simulink model "AWD_EV_MODEL_rev2"  (Simulink 8.7)
settings: Solver=ode3  SolverMode=SingleTasking  StartTime=0.0  StopTime=25  FixedStep=0.001  RelTol=1e-3
undefined symbols (not defined in the file): Bx, Bx_2, By, By_2, Cx, Cx_2, Cy, Cy_2, Dx, Dx_2, Dy, Dy_2, Ex, Ex_2, Ey, Ey_2, g, GRR, GRR_E, hg, Jw, Jz, Lf, Lr, Lw, m, r0, Rw, rx1, rx1_2, rx2, rx2_2, ry1, ry1_2, ry2, ry2_2, sigbuilder_block, Vx0, Vy0, wRL0
libraries: simulink x3
settings Model: Creator=ETLAB  LastModifiedBy=kschmutz
settings SolverCC: AlgebraicLoopSolver=LineSearch
settings DataIOCC: SignalLoggingSaveFormat=ModelDataLogs
settings OptimizationCC: ExpressionDepthLimit=2147483647
settings DebuggingCC: SolverPrmCheckMsg=warning  InheritedTsInSrcMsg=none  FcnCallInpInsideContextMsg=EnableAllAsWarning  StateNameClashWarn=warning
settings GRTTargetCC: CombineOutputUpdateFcns=off  GRTInterface=on

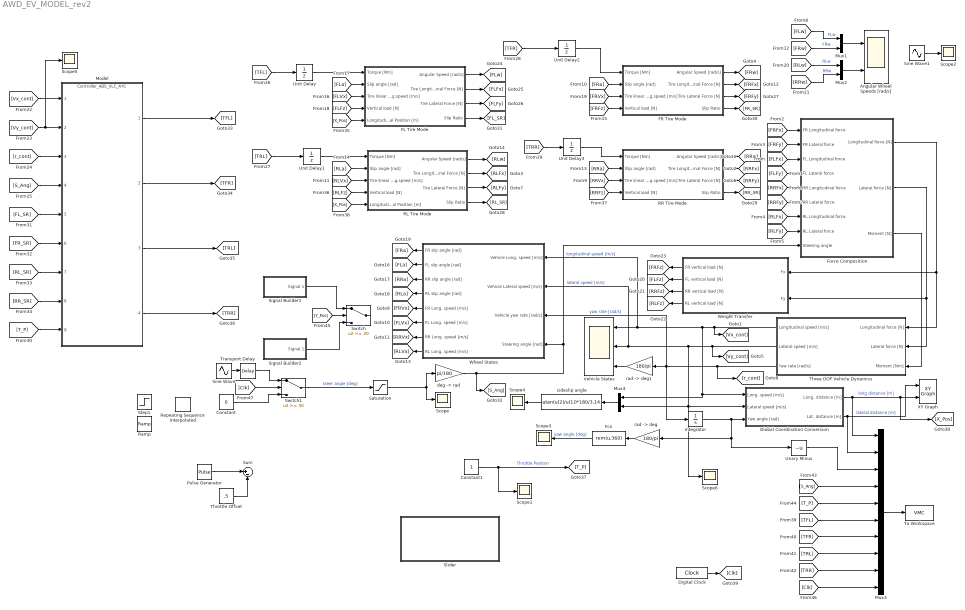
== system AWD_EV_MODEL_rev2 ==
  Angular Wheel Speeds [rad/s] : Scope  NumInputPorts=2
  Constant : Constant  Value=0
  Constant1 : Constant
  Digital Clock : DigitalClock  SampleTime=0.001
  FL Tire Mode : Subsystem
      mask Display:
      | image(imread('Tire.bmp'),'center')
      | port_label('input', 1, 'Torque [Nm]')
      | port_label('input', 2, 'Slip angle [rad]')
      | port_label('input', 3, 'Long. speed [m/s]')
      | port_label('input', 4, 'Vertical load [N]')
      | port_label('input', 5, 'Longitudinal Pos [m]')
      | port_label('output', 1, 'Angular speed [rad/s]')
      | port_label('output', 2, 'Long. force [N]')
      | port_label('output', 3, 'Lateral force [N]')
      | port_label('output', 4, 'Slip Ratio')
  FR Tire Mode : Subsystem
      mask Display:
      | image(imread('Tire.bmp'),'center')
      | port_label('input', 1, 'Torque [Nm]')
      | port_label('input', 2, 'Slip angle [rad]')
      | port_label('input', 3, 'Long. speed [m/s]')
      | port_label('input', 4, 'Vertical load [N]')
      | port_label('output', 1, 'Angular speed [rad/s]')
      | port_label('output', 2, 'Long. force [N]')
      | port_label('output', 3, 'Lateral force [N]')
      | port_label('output', 4, 'Slip Ratio')
  Fcn : Fcn  Expr=rem(u,360)
  Force Composition : Subsystem
  Global Coordination Conversion : Subsystem
  Integrator : Integrator
  Model : ModelReference  ModelNameDialog=Controller_ABS_VLC_AYC  SimulationMode=Normal  ModelReferenceVersion=1.127
  Mux1 : Mux  Inputs=2
  Mux2 : Mux  Inputs=2
  Mux3 : Mux  Inputs=10
  Mux4 : Mux  Inputs=2
  Pulse Generator : DiscretePulseGenerator  PulseType=Time based  Amplitude=.5  Period=7  PulseWidth=50
  RL Tire Mode : Subsystem
      mask Display:
      | image(imread('Tire.bmp'),'center')
      | port_label('input', 1, 'Torque [Nm]')
      | port_label('input', 2, 'Slip angle [rad]')
      | port_label('input', 3, 'Long. speed [m/s]')
      | port_label('input', 4, 'Vertical load [N]')
      | port_label('input', 5, 'Longitudinal Pos [m]')
      | port_label('output', 1, 'Angular speed [rad/s]')
      | port_label('output', 2, 'Long. force [N]')
      | port_label('output', 3, 'Lateral force [N]')
      | port_label('output', 4, 'Slip Ratio')
  RR Tire Mode : Subsystem
      mask Display:
      | image(imread('Tire.bmp'),'center')
      | port_label('input', 1, 'Torque [Nm]')
      | port_label('input', 2, 'Slip angle [rad]')
      | port_label('input', 3, 'Long. speed [m/s]')
      | port_label('input', 4, 'Vertical load [N]')
      | port_label('output', 1, 'Angular speed [rad/s]')
      | port_label('output', 2, 'Long. force [N]')
      | port_label('output', 3, 'Lateral force [N]')
  Ramp : simulink/Sources/Ramp  slope=0  start=.2  X0=0
  Repeating Sequence Interpolated : simulink/Sources/Repeating Sequence Interpolated  OutValues=[0 0 7 0 0 -7 0 0].'  TimeValues=[0 2 4 6 8 10 26 28].'  LookUpMeth=Interpolation-Use End Values  tsamp=0.001  OutMin=[]  OutMax=[]  OutDataTypeStr=double  OutputDataTypeScalingMode=double  OutDataType=fixdt(0,8)  OutScaling=2^-10
  Saturation : Saturate  UpperLimit=15  LowerLimit=-15
  Scope{,1..6} (7 alike) : Scope
  Signal Builder1 : Subsystem  Tag=STV Subsys  LoadFcn=sigbuilder_block('load');  StartFcn=sigbuilder_block('start');  StopFcn=sigbuilder_block('stop');  ClipboardFcn=sigbuilder_block('clipboard');  mask(Sigbuilder block){}
      mask help: Simulink:masks:SigbuilderBlock_MD
      mask init:
      | if ~strcmp(get_param(bdroot(gcbh),'SimulationStatus'),'stopped') tuvar = sigbuilder_block('maskInit'); end
      settings: CopyFcn=sigbuilder_block('copy');  DeleteFcn=sigbuilder_block('delete');  ModelCloseFcn=sigbuilder_block('modelClose');  PreSaveFcn=sigbuilder_block('preSave');  PauseFcn=sigbuilder_block('pause');  ContinueFcn=sigbuilder_block('continue');  NameChangeFcn=sigbuilder_block('namechange');  OpenFcn=sigbuilder_block('open',[6 36 1428 711 ]);  CloseFcn=sigbuilder_block('close');
      mask Display: plot(0, 0, 100, 100,[2, 2, 32, 32, 2], [68, 8, 8, 68, 68],[32, 2], [38, 38], [32, 19, 2],[53, 60, 44], [32, 17, 17, 2],[16, 16, 31, 31]);txt = getActiveGroup(gcbh);text(2, 100, txt,'verticalAlignment', 'top');
  Signal Builder2 : Subsystem  Tag=STV Subsys  LoadFcn=sigbuilder_block('load');  StartFcn=sigbuilder_block('start');  StopFcn=sigbuilder_block('stop');  ClipboardFcn=sigbuilder_block('clipboard');  mask(Sigbuilder block){}
      mask help: Simulink:masks:SigbuilderBlock_MD
      mask init:
      | if ~strcmp(get_param(bdroot(gcbh),'SimulationStatus'),'stopped') tuvar = sigbuilder_block('maskInit'); end
      settings: CopyFcn=sigbuilder_block('copy');  DeleteFcn=sigbuilder_block('delete');  ModelCloseFcn=sigbuilder_block('modelClose');  PreSaveFcn=sigbuilder_block('preSave');  PauseFcn=sigbuilder_block('pause');  ContinueFcn=sigbuilder_block('continue');  NameChangeFcn=sigbuilder_block('namechange');  OpenFcn=sigbuilder_block('open',[6 36 1428 711 ]);  CloseFcn=sigbuilder_block('close');
      mask Display: plot(0, 0, 100, 100,[2, 2, 32, 32, 2], [68, 8, 8, 68, 68],[32, 2], [38, 38], [32, 19, 2],[53, 60, 44], [32, 17, 17, 2],[16, 16, 31, 31]);txt = getActiveGroup(gcbh);text(2, 100, txt,'verticalAlignment', 'top');
  Sine Wave : Sin  Amplitude=4  Frequency=.1  SampleTime=0
  Sine Wave1 : Sin  Frequency=0.5  SampleTime=0
  Slider : Subsystem  DialogController=hmiCreateDDGDialog  DialogControllerArgs=DataTag4  IsWebBlock=on  mask(MWDashboardBlock){webBlockId=ca84606d-5772-4c84-acb2-69dff7348784, webBlockType=slider, ShowInLibBrowser=on, ShowInitialText=on, HMISrcModelName=AWD_EV_MODEL_rev2}
      mask prompts: webBlockId "WebBlock Id"; webBlockType "WebBlock Type"; HMISrcModelName "Source Model"
      mask Help: helpview([docroot '/mapfiles/simulink.map'], 'hmi_slider')
      mask Display:
      | if strcmp(get_param(bdroot(gcb),'BlockDiagramType'), 'library')
      |     image([(matlabroot) '/toolbox/simulink/hmi/icons/Slider.png']);
      | end
  Step1 : Step  Time=0  After=5  SampleTime=0
  Sum : Sum  Inputs=|+-
  Switch : Switch  Threshold=20
  Switch1 : Switch  Threshold=30
  Three DOF Vehicle Dynamics : Subsystem
      mask Display:
      | image(imread('Vehicle.bmp'),'center')
      | port_label('input', 1, 'Longitudinal force [N]')
      | port_label('input', 2, 'Lateral force [N]')
      | port_label('input', 3, 'Moment [Nm]')
      | port_label('output', 1, 'Longitudinal speed [m/s]')
      | port_label('output', 2, 'Lateral speed [m/s]')
      | port_label('output', 3, 'Yaw rate [rad/s]')
  Throttle Offset : Constant  Value=.5
  To Workspace : ToWorkspace  VariableName=VMC  SampleTime=-1
  Transport Delay : TransportDelay  DelayTime=4
  Unary Minus : UnaryMinus
  Unit Delay{,1..3} (4 alike) : UnitDelay  InitialCondition=1  SampleTime=-1
  Vehicle States : Scope  NumInputPorts=3
  Weight Transfer : Subsystem
  Wheel States : Subsystem
  XY Graph : simulink/Sinks/XY Graph  xmin=-500  xmax=500  ymin=-500  ymax=500  st=-1
  "deg -> rad" : Gain  Gain=pi/180
  "rad -> deg" : Gain  Gain=180/pi
  "rad -> deg1" : Gain  Gain=180/pi
  sideslip angle : Fcn  Expr=atan(u(2)/u(1))*180/3.14
  wires:
  Wheel States/5(FR Long. speed [m/s]) -> [FRVx]
  Wheel States/6(FL Long. speed [m/s]) -> [FLVx]
  Wheel States/7(RR Long. speed [m/s]) -> [RRVx]
  Wheel States/8(RL Long. speed [m/s]) -> [RLVx]
  Three DOF Vehicle Dynamics/3(Yaw rate [rad/s]) -> "rad -> deg1"/1, Wheel States/3(Vehicle yaw rate [rad/s]), Integrator/1, [r_cont]  "yaw rate [rad/s]"
  Three DOF Vehicle Dynamics/2(Lateral speed [m/s]) -> Wheel States/2(Vehicle Lateral speed [m/s]), Vehicle States/2, Global Coordination Conversion/2(Lateral speed [m/s]), Mux4/2, Scope6/1, [Vy_cont]  "lateral speed [m/s]"
  Three DOF Vehicle Dynamics/1(Longitudinal speed [m/s]) -> Wheel States/1(Vehicle Long. speed [m/s]), Vehicle States/1, Global Coordination Conversion/1(Long. speed [m/s]), Mux4/1, [Vx_cont]  "longitudinal speed [m/s]"
  Wheel States/1("FR slip angle [rad] ") -> [FRa]
  Wheel States/2("FL slip angle [rad] ") -> [FLa]
  Wheel States/3("RR slip angle [rad] ") -> [RRa]
  Wheel States/4("RL slip angle [rad] ") -> [RLa]
  Force Composition/1(Longitudinal force [N]) -> Weight Transfer/1(Fx), Three DOF Vehicle Dynamics/1(Longitudinal force [N])
  [FRFx] -> Force Composition/1(FR Longitudinal force)
  [FRFy] -> Force Composition/2(FR Lateral force)
  [FLFx] -> Force Composition/3(FL Longitudinal force)
  [FLFy] -> Force Composition/4(FL Lateral force)
  [RRFx] -> Force Composition/5(RR Longitudinal force)
  [RRFy] -> Force Composition/6(RR Lateral force)
  [RLFx] -> Force Composition/7(RL Longitudinal force)
  [RLFy] -> Force Composition/8(RL Lateral force)
  "rad -> deg"/1 -> Fcn/1
  Fcn/1 -> Scope3/1  "yaw angle [deg]"
  Global Coordination Conversion/1(Long. distance [m]) -> Mux3/1, XY Graph/2, [X_Pos]  "long distance [m]"
  Global Coordination Conversion/2(Lat. distance [m]) -> XY Graph/1, Mux3/2  "lateral distance [m]"
  Weight Transfer/1(FR vertical load [N]) -> [FRFz]
  Weight Transfer/2(FL vertical load [N]) -> [FLFz]
  Weight Transfer/3(RR vertical load [N]) -> [RRFz]
  Weight Transfer/4(RL vertical load [N]) -> [RLFz]
  Force Composition/2(Lateral force [N]) -> Weight Transfer/2(Fy), Three DOF Vehicle Dynamics/2(Lateral force [N])
  Integrator/1 -> Global Coordination Conversion/3(Yaw angle [rad]), "rad -> deg"/1, Unary Minus/1
  Force Composition/3(Moment [N]) -> Three DOF Vehicle Dynamics/3(Moment [Nm])
  "rad -> deg1"/1 -> Vehicle States/3
  Mux4/1 -> sideslip angle/1
  sideslip angle/1 -> Scope4/1
  Sine Wave1/1 -> Scope2/1
  FL Tire Mode/2(Tire Longitudinal Force [N]) -> [FLFx]
  FL Tire Mode/1(Angular Speed [rad/s]) -> [FLw]
  [FLVx] -> FL Tire Mode/3(Tire linear Long.speed [m/s])
  [FLa] -> FL Tire Mode/2(Slip angle [rad])
  [FLFz] -> FL Tire Mode/4(Vertical load [N])
  FL Tire Mode/3(Tire Lateral Force [N]) -> [FLFy]
  [FLw] -> Mux1/1  "FLw"
  [FRw] -> Mux1/2  "FRw"
  [RLw] -> Mux2/1  "RLw"
  [RRw] -> Mux2/2  "RRw"
  Mux1/1 -> Angular Wheel Speeds [rad/s]/1
  Mux2/1 -> Angular Wheel Speeds [rad/s]/2
  FL Tire Mode/4(Slip Ratio) -> [FL_SR]
  Mux3/1 -> To Workspace/1
  [FRa] -> FR Tire Mode/2(Slip angle [rad])
  [FRVx] -> FR Tire Mode/3(Tire linear Long.speed [m/s])
  [FRFz] -> FR Tire Mode/4(Vertical load [N])
  FR Tire Mode/1(Angular Speed [rad/s]) -> [FRw]
  FR Tire Mode/2(Tire Longitudinal Force [N]) -> [FRFx]
  FR Tire Mode/3(Tire Lateral Force [N]) -> [FRFy]
  FR Tire Mode/4(Slip Ratio) -> [FR_SR]
  [RLa] -> RL Tire Mode/2(Slip angle [rad])
  [RLVx] -> RL Tire Mode/3(Tire linear Long.speed [m/s])
  [RLFz] -> RL Tire Mode/4(Vertical load [N])
  RL Tire Mode/1(Angular Speed [rad/s]) -> [RLw]
  RL Tire Mode/2(Tire Longitudinal Force [N]) -> [RLFx]
  RL Tire Mode/3(Tire Lateral Force [N]) -> [RLFy]
  RL Tire Mode/4(Slip Ratio) -> [RL_SR]
  [RRa] -> RR Tire Mode/2(Slip angle [rad])
  [RRVx] -> RR Tire Mode/3(Tire linear Long.speed [m/s])
  [RRFz] -> RR Tire Mode/4(Vertical load [N])
  RR Tire Mode/1(Angular Speed [rad/s]) -> [RRw]
  RR Tire Mode/2(Tire Longitudinal Force [N]) -> [RRFx]
  RR Tire Mode/3(Tire Lateral Force [N]) -> [RRFy]
  RR Tire Mode/4(Slip Ratio) -> [RR_SR]
  "deg -> rad"/1 -> [S_Ang], Wheel States/4(Steering angle [rad]), Force Composition/9(Steering angle)
  Switch1/1 -> Saturation/1  "steer angle [deg]"
  Saturation/1 -> "deg -> rad"/1, Scope/1
  Unary Minus/1 -> Mux3/3
  Constant1/1 -> Scope1/1, [T_P]  "Throttle Position"
  Pulse Generator/1 -> Sum/1
  Throttle Offset/1 -> Sum/2
  [Vx_cont] -> Model/1
  [Vy_cont] -> Model/2, Scope5/1
  [r_cont] -> Model/3
  [S_Ang] -> Model/4
  [FL_SR] -> Model/5
  [FR_SR] -> Model/6
  [RL_SR] -> Model/7
  [RR_SR] -> Model/8
  [T_P] -> Model/9
  [X_Pos] -> FL Tire Mode/5(Longitudinal Position [m])
  [X_Pos] -> RL Tire Mode/5(Longitudinal Position [m])
  [S_Ang] -> Mux3/4
  [TFL] -> Mux3/6
  [TFR] -> Mux3/7
  [TRL] -> Mux3/8
  [TRR] -> Mux3/9
  [T_P] -> Mux3/5
  [Clk] -> Mux3/10
  [TFR] -> Unit Delay2/1
  [TRR] -> Unit Delay3/1
  [TRL] -> Unit Delay1/1
  [TFL] -> Unit Delay/1
  [Y_Pos] -> Switch/2
  Signal Builder1/1(Signal 1) -> Switch/1
  Signal Builder2/1(Signal 1) -> Switch/3
  Digital Clock/1 -> [Clk]
  [Clk] -> Switch1/2
  Sine Wave/1 -> Transport Delay/1
  Constant/1 -> Switch1/3
  Transport Delay/1 -> Switch1/1
  Model/1 -> [TFL]
  Model/2 -> [TFR]
  Model/3 -> [TRL]
  Model/4 -> [TRR]
  Unit Delay/1 -> FL Tire Mode/1(Torque [Nm])
  Unit Delay3/1 -> RR Tire Mode/1(Torque [Nm])
  Unit Delay1/1 -> RL Tire Mode/1(Torque [Nm])
  Unit Delay2/1 -> FR Tire Mode/1(Torque [Nm])

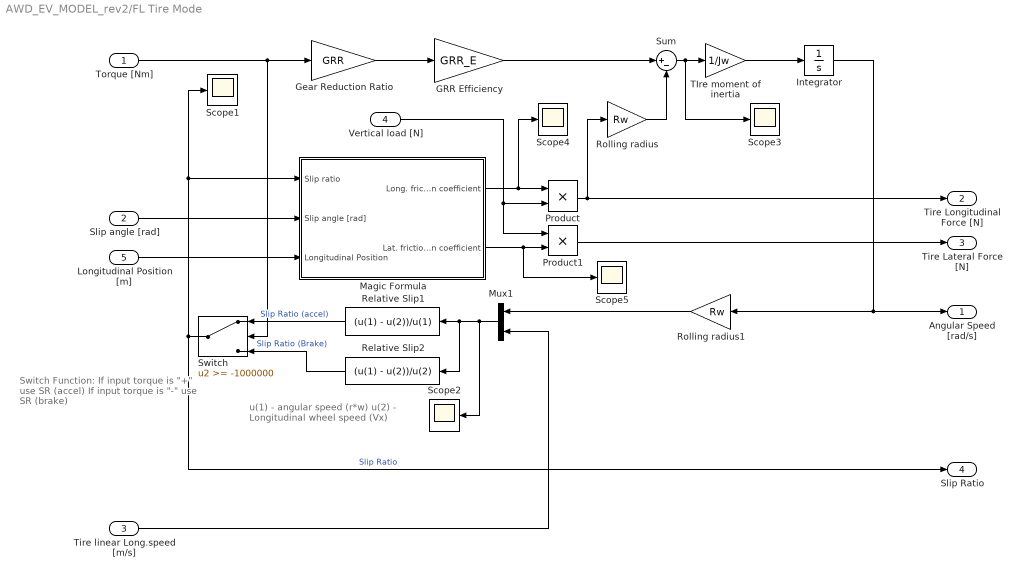
== system AWD_EV_MODEL_rev2/FL Tire Mode ==
  note: u(1) - angular speed (r*w)
      | u(2) - Longitudinal wheel speed (Vx)
  note: Switch Function:
      | If input torque is "+" use SR (accel)
      | If input torque is "-" use SR (brake)
  Torque [Nm] : Inport
  Slip angle [rad] : Inport  Port=2
  Tire linear Long.speed [m/s] : Inport  Port=3
  Vertical load [N] : Inport  Port=4
  Longitudinal Position [m] : Inport  Port=5
  GRR Efficiency : Gain  Gain=GRR_E  SaturateOnIntegerOverflow=on  OutDataTypeStr=Inherit: Same as input  ParamDataTypeStr=Inherit: Same as input
  Gear Reduction Ratio : Gain  Gain=GRR  SaturateOnIntegerOverflow=on  OutDataTypeStr=Inherit: Same as input  ParamDataTypeStr=Inherit: Same as input
  Integrator : Integrator  InitialCondition=wRL0
  Magic Formula : Subsystem  mask(Magic Formula (Combined Slip)){}
      mask Display:
      | image(imread('Magic formula.jpg'),'center')
      | port_label('input', 1, 'slip ratio')
      | port_label('input', 2, 'slip angle')
      | port_label('output', 1, 'Mux')
      | port_label('output', 2, 'Muy')
  Mux1 : Mux  Inputs=2
  Product : Product  RndMeth=Zero
  Product1 : Product  RndMeth=Zero
  Relative Slip1 : Fcn  Expr=(u(1) - u(2))/u(1)
  Relative Slip2 : Fcn  Expr=(u(1) - u(2))/u(2)
  Rolling radius : Gain  Gain=Rw  SaturateOnIntegerOverflow=on  OutDataTypeStr=Inherit: Same as input  ParamDataTypeStr=Inherit: Same as input
  Rolling radius1 : Gain  Gain=Rw  SaturateOnIntegerOverflow=on  OutDataTypeStr=Inherit: Same as input  ParamDataTypeStr=Inherit: Same as input
  Scope{1..5} (5 alike) : Scope
  Sum : Sum  Inputs=|+-
  Switch : Switch  Threshold=-1000000
  TIre moment of inertia : Gain  Gain=1/Jw  SaturateOnIntegerOverflow=on  OutDataTypeStr=Inherit: Same as input  ParamDataTypeStr=Inherit: Same as input
  Angular Speed [rad/s] : Outport
  Tire Longitudinal Force [N] : Outport  Port=2
  Tire Lateral Force [N] : Outport  Port=3
  Slip Ratio : Outport  Port=4
  wires:
  Slip angle [rad]/1 -> Magic Formula/2(Slip angle [rad])
  Tire linear Long.speed [m/s]/1 -> Mux1/2
  Torque [Nm]/1 -> Gear Reduction Ratio/1, Switch/2
  Sum/1 -> TIre moment of inertia/1, Scope3/1
  TIre moment of inertia/1 -> Integrator/1
  Integrator/1 -> Angular Speed [rad/s]/1, Rolling radius1/1
  Rolling radius/1 -> Sum/2
  Mux1/1 -> Scope2/1, Relative Slip1/1, Relative Slip2/1
  Rolling radius1/1 -> Mux1/1
  Magic Formula/1(Long. friction coefficient) -> Product/1, Scope4/1
  Magic Formula/2(Lat. friction coefficient) -> Product1/2, Scope5/1
  Product/1 -> Rolling radius/1, Tire Longitudinal Force [N]/1
  Vertical load [N]/1 -> Product/2, Product1/1
  Product1/1 -> Tire Lateral Force [N]/1
  Gear Reduction Ratio/1 -> GRR Efficiency/1
  GRR Efficiency/1 -> Sum/1
  Relative Slip1/1 -> Switch/1  "Slip Ratio (accel)"
  Relative Slip2/1 -> Switch/3  "Slip Ratio (Brake)"
  Switch/1 -> Magic Formula/1(Slip ratio), Scope1/1, Slip Ratio/1  "Slip Ratio"
  Longitudinal Position [m]/1 -> Magic Formula/3(Longitudinal Position)

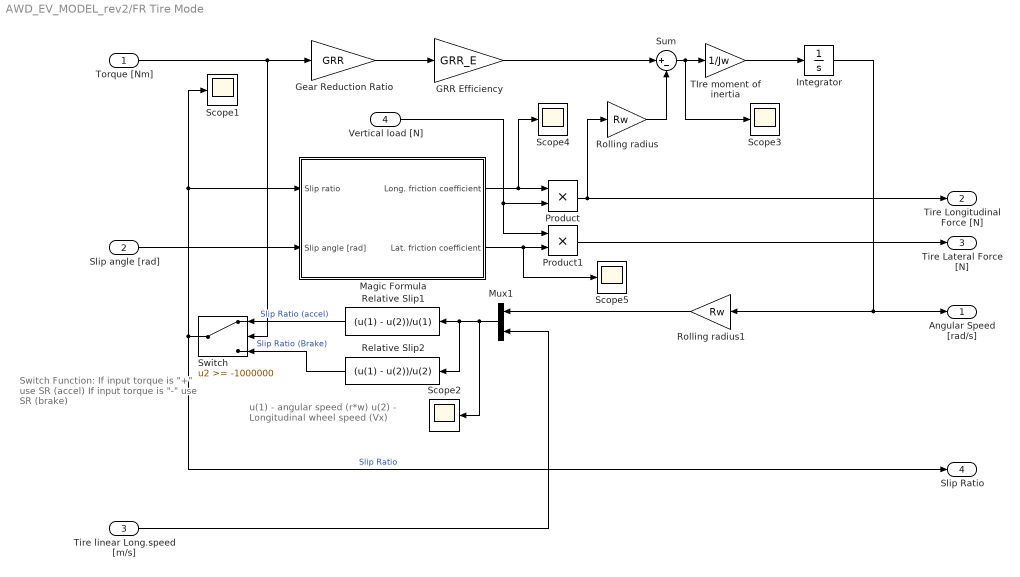
== system AWD_EV_MODEL_rev2/FR Tire Mode ==
  note: u(1) - angular speed (r*w)
      | u(2) - Longitudinal wheel speed (Vx)
  note: Switch Function:
      | If input torque is "+" use SR (accel)
      | If input torque is "-" use SR (brake)
  Torque [Nm] : Inport
  Slip angle [rad] : Inport  Port=2
  Tire linear Long.speed [m/s] : Inport  Port=3
  Vertical load [N] : Inport  Port=4
  GRR Efficiency : Gain  Gain=GRR_E  SaturateOnIntegerOverflow=on  OutDataTypeStr=Inherit: Same as input  ParamDataTypeStr=Inherit: Same as input
  Gear Reduction Ratio : Gain  Gain=GRR  SaturateOnIntegerOverflow=on  OutDataTypeStr=Inherit: Same as input  ParamDataTypeStr=Inherit: Same as input
  Integrator : Integrator  InitialCondition=wRL0
  Magic Formula : Subsystem  mask(Magic Formula (Combined Slip)){}
      mask Display:
      | image(imread('Magic formula.jpg'),'center')
      | port_label('input', 1, 'slip ratio')
      | port_label('input', 2, 'slip angle')
      | port_label('output', 1, 'Mux')
      | port_label('output', 2, 'Muy')
  Mux1 : Mux  Inputs=2
  Product : Product  RndMeth=Zero
  Product1 : Product  RndMeth=Zero
  Relative Slip1 : Fcn  Expr=(u(1) - u(2))/u(1)
  Relative Slip2 : Fcn  Expr=(u(1) - u(2))/u(2)
  Rolling radius : Gain  Gain=Rw  SaturateOnIntegerOverflow=on  OutDataTypeStr=Inherit: Same as input  ParamDataTypeStr=Inherit: Same as input
  Rolling radius1 : Gain  Gain=Rw  SaturateOnIntegerOverflow=on  OutDataTypeStr=Inherit: Same as input  ParamDataTypeStr=Inherit: Same as input
  Scope{1..5} (5 alike) : Scope
  Sum : Sum  Inputs=|+-
  Switch : Switch  Threshold=-1000000
  TIre moment of inertia : Gain  Gain=1/Jw  SaturateOnIntegerOverflow=on  OutDataTypeStr=Inherit: Same as input  ParamDataTypeStr=Inherit: Same as input
  Angular Speed [rad/s] : Outport
  Tire Longitudinal Force [N] : Outport  Port=2
  Tire Lateral Force [N] : Outport  Port=3
  Slip Ratio : Outport  Port=4
  wires:
  Slip angle [rad]/1 -> Magic Formula/2(Slip angle [rad])
  Tire linear Long.speed [m/s]/1 -> Mux1/2
  Torque [Nm]/1 -> Gear Reduction Ratio/1, Switch/2
  Sum/1 -> TIre moment of inertia/1, Scope3/1
  TIre moment of inertia/1 -> Integrator/1
  Integrator/1 -> Angular Speed [rad/s]/1, Rolling radius1/1
  Rolling radius/1 -> Sum/2
  Mux1/1 -> Scope2/1, Relative Slip1/1, Relative Slip2/1
  Rolling radius1/1 -> Mux1/1
  Magic Formula/1(Long. friction coefficient) -> Product/1, Scope4/1
  Magic Formula/2(Lat. friction coefficient) -> Product1/2, Scope5/1
  Product/1 -> Rolling radius/1, Tire Longitudinal Force [N]/1
  Vertical load [N]/1 -> Product/2, Product1/1
  Product1/1 -> Tire Lateral Force [N]/1
  Gear Reduction Ratio/1 -> GRR Efficiency/1
  GRR Efficiency/1 -> Sum/1
  Relative Slip1/1 -> Switch/1  "Slip Ratio (accel)"
  Relative Slip2/1 -> Switch/3  "Slip Ratio (Brake)"
  Switch/1 -> Magic Formula/1(Slip ratio), Scope1/1, Slip Ratio/1  "Slip Ratio"

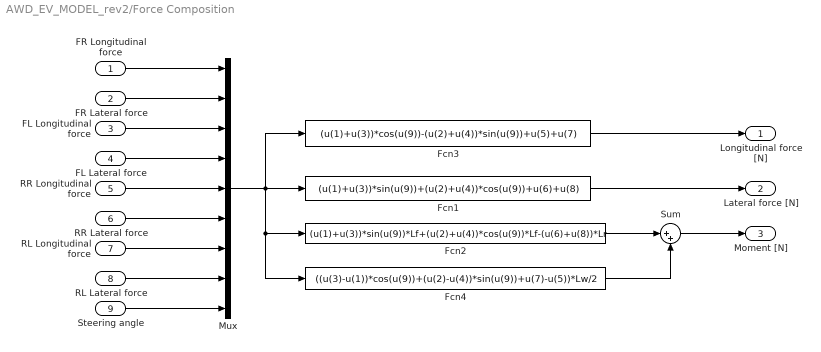
== system AWD_EV_MODEL_rev2/Force Composition ==
  FR Longitudinal force : Inport
  FR Lateral force : Inport  Port=2
  FL Longitudinal force : Inport  Port=3
  FL Lateral force : Inport  Port=4
  RR Longitudinal force : Inport  Port=5
  RR Lateral force : Inport  Port=6
  RL Longitudinal force : Inport  Port=7
  RL Lateral force : Inport  Port=8
  Steering angle : Inport  Port=9
  Fcn1 : Fcn  Expr=(u(1)+u(3))*sin(u(9))+(u(2)+u(4))*cos(u(9))+u(6)+u(8)
  Fcn2 : Fcn  Expr=(u(1)+u(3))*sin(u(9))*Lf+(u(2)+u(4))*cos(u(9))*Lf-(u(6)+u(8))*Lr
  Fcn3 : Fcn  Expr=(u(1)+u(3))*cos(u(9))-(u(2)+u(4))*sin(u(9))+u(5)+u(7)
  Fcn4 : Fcn  Expr=((u(3)-u(1))*cos(u(9))+(u(2)-u(4))*sin(u(9))+u(7)-u(5))*Lw/2
  Mux : Mux  Inputs=9
  Sum : Sum  Inputs=|++
  Longitudinal force [N] : Outport
  Lateral force [N] : Outport  Port=2
  Moment [N] : Outport  Port=3
  wires:
  Mux/1 -> Fcn3/1, Fcn1/1, Fcn2/1, Fcn4/1
  Fcn3/1 -> Longitudinal force [N]/1
  Fcn1/1 -> Lateral force [N]/1
  Sum/1 -> Moment [N]/1
  Fcn2/1 -> Sum/1
  Fcn4/1 -> Sum/2
  FR Longitudinal force/1 -> Mux/1
  FR Lateral force/1 -> Mux/2
  FL Longitudinal force/1 -> Mux/3
  FL Lateral force/1 -> Mux/4
  RR Longitudinal force/1 -> Mux/5
  RR Lateral force/1 -> Mux/6
  RL Longitudinal force/1 -> Mux/7
  RL Lateral force/1 -> Mux/8
  Steering angle/1 -> Mux/9

== system AWD_EV_MODEL_rev2/Global Coordination Conversion ==
  Long. speed [m/s] : Inport
  Lateral speed [m/s] : Inport  Port=2
  Yaw angle [rad] : Inport  Port=3
  Fcn : Fcn  Expr=cos(u(3))*u(1)-sin(u(3))*u(2)
  Fcn1 : Fcn  Expr=sin(u(3))*u(1)+cos(u(3))*u(2)
  Integrator : Integrator
  Integrator1 : Integrator
  Mux : Mux  Inputs=3
  Long. distance [m] : Outport
  Lat. distance [m] : Outport  Port=2
  wires:
  Long. speed [m/s]/1 -> Mux/1
  Lateral speed [m/s]/1 -> Mux/2
  Yaw angle [rad]/1 -> Mux/3
  Mux/1 -> Fcn/1, Fcn1/1
  Fcn/1 -> Integrator/1
  Fcn1/1 -> Integrator1/1
  Integrator/1 -> Long. distance [m]/1
  Integrator1/1 -> Lat. distance [m]/1

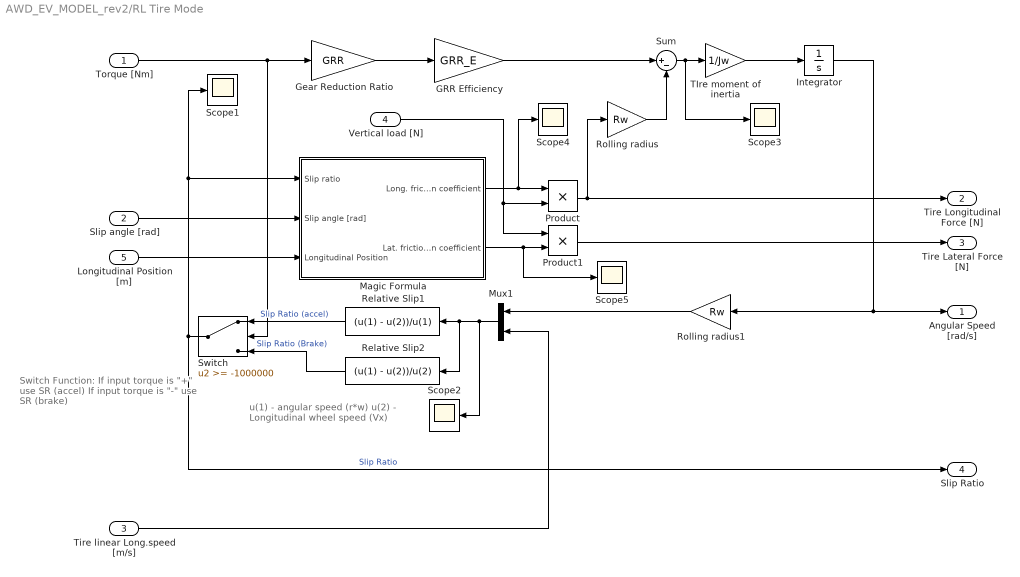
== system AWD_EV_MODEL_rev2/RL Tire Mode ==
  note: u(1) - angular speed (r*w)
      | u(2) - Longitudinal wheel speed (Vx)
  note: Switch Function:
      | If input torque is "+" use SR (accel)
      | If input torque is "-" use SR (brake)
  Torque [Nm] : Inport
  Slip angle [rad] : Inport  Port=2
  Tire linear Long.speed [m/s] : Inport  Port=3
  Vertical load [N] : Inport  Port=4
  Longitudinal Position [m] : Inport  Port=5
  GRR Efficiency : Gain  Gain=GRR_E  SaturateOnIntegerOverflow=on  OutDataTypeStr=Inherit: Same as input  ParamDataTypeStr=Inherit: Same as input
  Gear Reduction Ratio : Gain  Gain=GRR  SaturateOnIntegerOverflow=on  OutDataTypeStr=Inherit: Same as input  ParamDataTypeStr=Inherit: Same as input
  Integrator : Integrator  InitialCondition=wRL0
  Magic Formula : Subsystem  mask(Magic Formula (Combined Slip)){}
      mask Display:
      | image(imread('Magic formula.jpg'),'center')
      | port_label('input', 1, 'slip ratio')
      | port_label('input', 2, 'slip angle')
      | port_label('output', 1, 'Mux')
      | port_label('output', 2, 'Muy')
  Mux1 : Mux  Inputs=2
  Product : Product  RndMeth=Zero
  Product1 : Product  RndMeth=Zero
  Relative Slip1 : Fcn  Expr=(u(1) - u(2))/u(1)
  Relative Slip2 : Fcn  Expr=(u(1) - u(2))/u(2)
  Rolling radius : Gain  Gain=Rw  SaturateOnIntegerOverflow=on  OutDataTypeStr=Inherit: Same as input  ParamDataTypeStr=Inherit: Same as input
  Rolling radius1 : Gain  Gain=Rw  SaturateOnIntegerOverflow=on  OutDataTypeStr=Inherit: Same as input  ParamDataTypeStr=Inherit: Same as input
  Scope{1..5} (5 alike) : Scope
  Sum : Sum  Inputs=|+-
  Switch : Switch  Threshold=-1000000
  TIre moment of inertia : Gain  Gain=1/Jw  SaturateOnIntegerOverflow=on  OutDataTypeStr=Inherit: Same as input  ParamDataTypeStr=Inherit: Same as input
  Angular Speed [rad/s] : Outport
  Tire Longitudinal Force [N] : Outport  Port=2
  Tire Lateral Force [N] : Outport  Port=3
  Slip Ratio : Outport  Port=4
  wires:
  Slip angle [rad]/1 -> Magic Formula/2(Slip angle [rad])
  Tire linear Long.speed [m/s]/1 -> Mux1/2
  Torque [Nm]/1 -> Gear Reduction Ratio/1, Switch/2
  Sum/1 -> TIre moment of inertia/1, Scope3/1
  TIre moment of inertia/1 -> Integrator/1
  Integrator/1 -> Angular Speed [rad/s]/1, Rolling radius1/1
  Rolling radius/1 -> Sum/2
  Mux1/1 -> Scope2/1, Relative Slip1/1, Relative Slip2/1
  Rolling radius1/1 -> Mux1/1
  Magic Formula/1(Long. friction coefficient) -> Product/1, Scope4/1
  Magic Formula/2(Lat. friction coefficient) -> Product1/2, Scope5/1
  Product/1 -> Rolling radius/1, Tire Longitudinal Force [N]/1
  Vertical load [N]/1 -> Product/2, Product1/1
  Product1/1 -> Tire Lateral Force [N]/1
  Gear Reduction Ratio/1 -> GRR Efficiency/1
  GRR Efficiency/1 -> Sum/1
  Relative Slip1/1 -> Switch/1  "Slip Ratio (accel)"
  Relative Slip2/1 -> Switch/3  "Slip Ratio (Brake)"
  Switch/1 -> Magic Formula/1(Slip ratio), Scope1/1, Slip Ratio/1  "Slip Ratio"
  Longitudinal Position [m]/1 -> Magic Formula/3(Longitudinal Position)

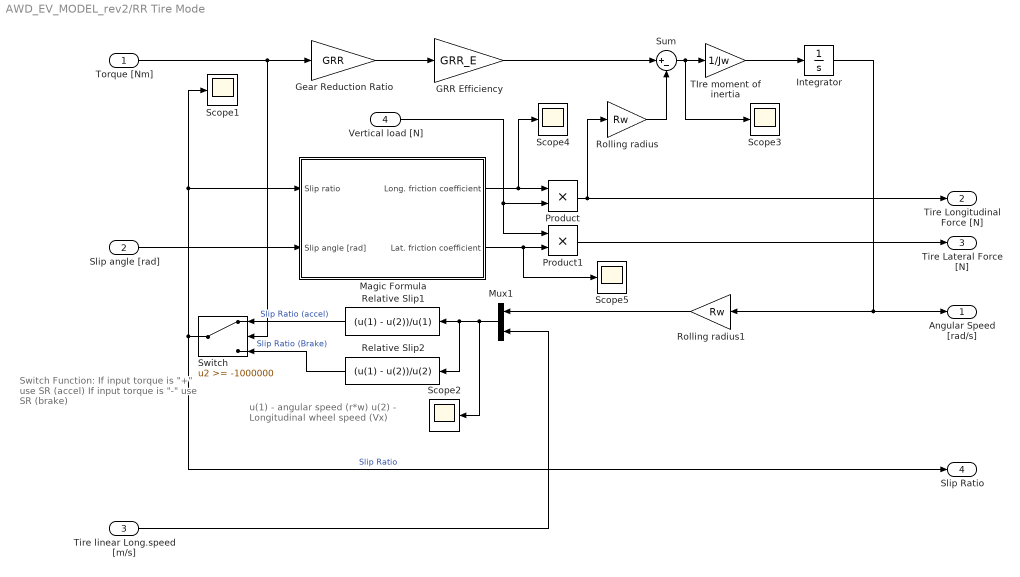
== system AWD_EV_MODEL_rev2/RR Tire Mode ==
  note: u(1) - angular speed (r*w)
      | u(2) - Longitudinal wheel speed (Vx)
  note: Switch Function:
      | If input torque is "+" use SR (accel)
      | If input torque is "-" use SR (brake)
  Torque [Nm] : Inport
  Slip angle [rad] : Inport  Port=2
  Tire linear Long.speed [m/s] : Inport  Port=3
  Vertical load [N] : Inport  Port=4
  GRR Efficiency : Gain  Gain=GRR_E  SaturateOnIntegerOverflow=on  OutDataTypeStr=Inherit: Same as input  ParamDataTypeStr=Inherit: Same as input
  Gear Reduction Ratio : Gain  Gain=GRR  SaturateOnIntegerOverflow=on  OutDataTypeStr=Inherit: Same as input  ParamDataTypeStr=Inherit: Same as input
  Integrator : Integrator  InitialCondition=wRL0
  Magic Formula : Subsystem  mask(Magic Formula (Combined Slip)){}
      mask Display:
      | image(imread('Magic formula.jpg'),'center')
      | port_label('input', 1, 'slip ratio')
      | port_label('input', 2, 'slip angle')
      | port_label('output', 1, 'Mux')
      | port_label('output', 2, 'Muy')
  Mux1 : Mux  Inputs=2
  Product : Product  RndMeth=Zero
  Product1 : Product  RndMeth=Zero
  Relative Slip1 : Fcn  Expr=(u(1) - u(2))/u(1)
  Relative Slip2 : Fcn  Expr=(u(1) - u(2))/u(2)
  Rolling radius : Gain  Gain=Rw  SaturateOnIntegerOverflow=on  OutDataTypeStr=Inherit: Same as input  ParamDataTypeStr=Inherit: Same as input
  Rolling radius1 : Gain  Gain=Rw  SaturateOnIntegerOverflow=on  OutDataTypeStr=Inherit: Same as input  ParamDataTypeStr=Inherit: Same as input
  Scope{1..5} (5 alike) : Scope
  Sum : Sum  Inputs=|+-
  Switch : Switch  Threshold=-1000000
  TIre moment of inertia : Gain  Gain=1/Jw  SaturateOnIntegerOverflow=on  OutDataTypeStr=Inherit: Same as input  ParamDataTypeStr=Inherit: Same as input
  Angular Speed [rad/s] : Outport
  Tire Longitudinal Force [N] : Outport  Port=2
  Tire Lateral Force [N] : Outport  Port=3
  Slip Ratio : Outport  Port=4
  wires:
  Slip angle [rad]/1 -> Magic Formula/2(Slip angle [rad])
  Tire linear Long.speed [m/s]/1 -> Mux1/2
  Torque [Nm]/1 -> Gear Reduction Ratio/1, Switch/2
  Sum/1 -> TIre moment of inertia/1, Scope3/1
  TIre moment of inertia/1 -> Integrator/1
  Integrator/1 -> Angular Speed [rad/s]/1, Rolling radius1/1
  Rolling radius/1 -> Sum/2
  Mux1/1 -> Scope2/1, Relative Slip1/1, Relative Slip2/1
  Rolling radius1/1 -> Mux1/1
  Magic Formula/1(Long. friction coefficient) -> Product/1, Scope4/1
  Magic Formula/2(Lat. friction coefficient) -> Product1/2, Scope5/1
  Product/1 -> Rolling radius/1, Tire Longitudinal Force [N]/1
  Vertical load [N]/1 -> Product/2, Product1/1
  Product1/1 -> Tire Lateral Force [N]/1
  Gear Reduction Ratio/1 -> GRR Efficiency/1
  GRR Efficiency/1 -> Sum/1
  Relative Slip1/1 -> Switch/1  "Slip Ratio (accel)"
  Relative Slip2/1 -> Switch/3  "Slip Ratio (Brake)"
  Switch/1 -> Magic Formula/1(Slip ratio), Scope1/1, Slip Ratio/1  "Slip Ratio"

== system AWD_EV_MODEL_rev2/Signal Builder1 ==
  Demux : Demux  Tag=STV Demux  Outputs=1
  FromWs : FromWorkspace  Tag=STV FromWs  VariableName=tuvar  SampleTime=0  SigBuilderData=DataTag0  VnvData=DataTag1
      SigBuilderData=|
      | common.afterFinalStr = 'Extrapolate'
      | common.sampleTime = 0
      | dataSet.timeRange = [0 15]
      | dataSet.name = 'Group 1'
      | sbobj.Groups.Name = 'Group 1'
      | sbobj.Groups.Signals.Name = 'Signal 1'
      | sbobj.Groups.Signals.XData = [0 1.99 15]
      | sbobj.Groups.Signals.YData = [9.9 -10.05 -9.95]
      | sbobj.Groups.TimeRange = [0 15]
  Signal 1 : Outport  Tag=STV Outport
  wires:
  Demux/1 -> Signal 1/1
  FromWs/1 -> Demux/1

== system AWD_EV_MODEL_rev2/Signal Builder2 ==
  Demux : Demux  Tag=STV Demux  Outputs=1
  FromWs : FromWorkspace  Tag=STV FromWs  VariableName=tuvar  SampleTime=0  SigBuilderData=DataTag2  VnvData=DataTag3
      SigBuilderData=|
      | common.afterFinalStr = 'Extrapolate'
      | common.sampleTime = 0
      | dataSet.timeRange = [0 15]
      | dataSet.name = 'Group 1'
      | sbobj.Groups.Name = 'Group 1'
      | sbobj.Groups.Signals.Name = 'Signal 1'
      | sbobj.Groups.Signals.XData = [0 1.99 15]
      | sbobj.Groups.Signals.YData = [-10.05 10 10]
      | sbobj.Groups.TimeRange = [0 15]
  Signal 1 : Outport  Tag=STV Outport
  wires:
  Demux/1 -> Signal 1/1
  FromWs/1 -> Demux/1

== system AWD_EV_MODEL_rev2/Slider ==

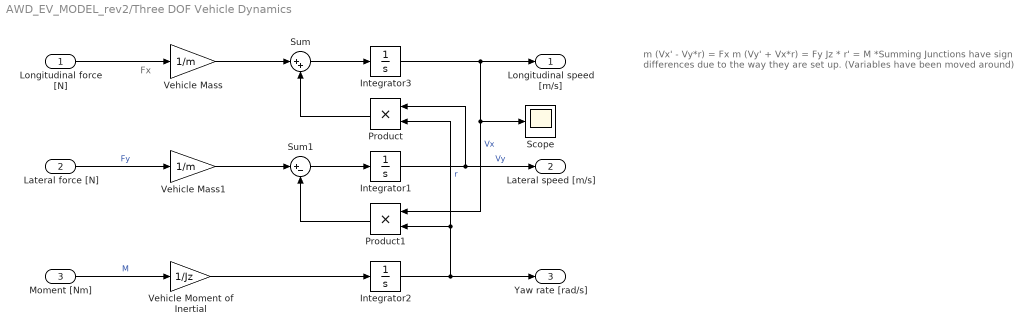
== system AWD_EV_MODEL_rev2/Three DOF Vehicle Dynamics ==
  note: m (Vx' - Vy*r) = Fx
      | m (Vy' + Vx*r) = Fy
      |
      | Jz * r' = M
      |
      | *Summing Junctions have sign differences due to
      | the way they are set up. (Variables have been moved around)
  note: Fx
  Longitudinal force [N] : Inport
  Lateral force [N] : Inport  Port=2
  Moment [Nm] : Inport  Port=3
  Integrator1 : Integrator  InitialCondition=Vy0  UpperSaturationLimit=1000  LowerSaturationLimit=0
  Integrator2 : Integrator  InitialCondition=r0
  Integrator3 : Integrator  InitialCondition=Vx0  UpperSaturationLimit=1000  LowerSaturationLimit=0
  Product : Product  RndMeth=Zero
  Product1 : Product  RndMeth=Zero
  Scope : Scope
  Sum : Sum  Inputs=|++
  Sum1 : Sum  Inputs=|+-
  Vehicle Mass : Gain  Gain=1/m
  Vehicle Mass1 : Gain  Gain=1/m
  Vehicle Moment of Inertial : Gain  Gain=1/Jz
  Longitudinal speed [m/s] : Outport
  Lateral speed [m/s] : Outport  Port=2
  Yaw rate [rad/s] : Outport  Port=3
  wires:
  Integrator2/1 -> Yaw rate [rad/s]/1, Product/2, Product1/2  "r"
  Moment [Nm]/1 -> Vehicle Moment of Inertial/1  "M"
  Integrator1/1 -> Product/1, Lateral speed [m/s]/1  "Vy"
  Integrator3/1 -> Longitudinal speed [m/s]/1, Product1/1, Scope/1  "Vx"
  Vehicle Moment of Inertial/1 -> Integrator2/1
  Vehicle Mass1/1 -> Sum1/1
  Lateral force [N]/1 -> Vehicle Mass1/1  "Fy"
  Vehicle Mass/1 -> Sum/1
  Sum1/1 -> Integrator1/1
  Product1/1 -> Sum1/2
  Sum/1 -> Integrator3/1
  Product/1 -> Sum/2
  Longitudinal force [N]/1 -> Vehicle Mass/1

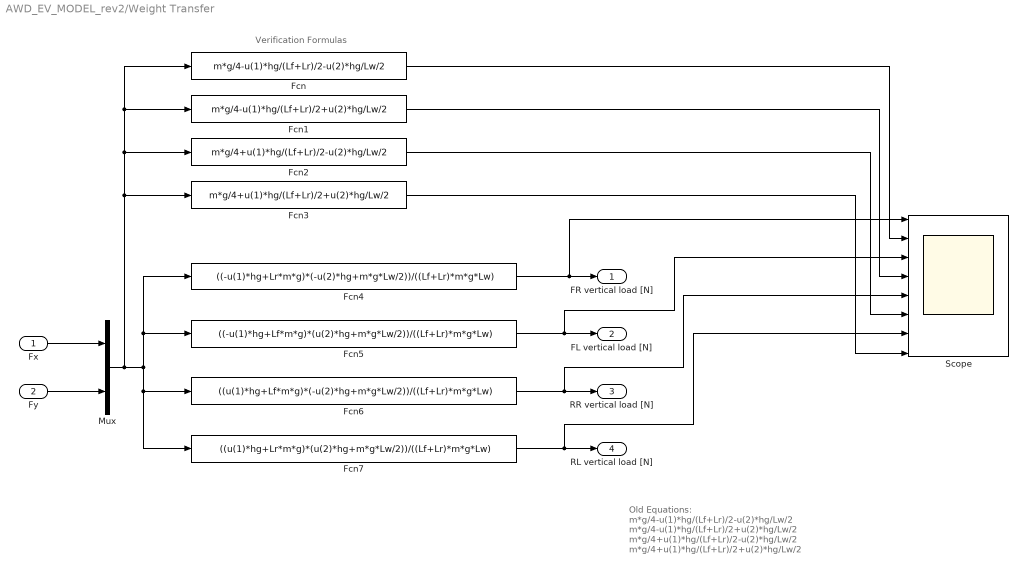
== system AWD_EV_MODEL_rev2/Weight Transfer ==
  note: Old Equations:
      | m*g/4-u(1)*hg/(Lf+Lr)/2-u(2)*hg/Lw/2
      | m*g/4-u(1)*hg/(Lf+Lr)/2+u(2)*hg/Lw/2
      | m*g/4+u(1)*hg/(Lf+Lr)/2-u(2)*hg/Lw/2
      | m*g/4+u(1)*hg/(Lf+Lr)/2+u(2)*hg/Lw/2
  note: Verification Formulas
  Fx : Inport
  Fy : Inport  Port=2
  Fcn : Fcn  Expr=m*g/4-u(1)*hg/(Lf+Lr)/2-u(2)*hg/Lw/2
  Fcn1 : Fcn  Expr=m*g/4-u(1)*hg/(Lf+Lr)/2+u(2)*hg/Lw/2
  Fcn2 : Fcn  Expr=m*g/4+u(1)*hg/(Lf+Lr)/2-u(2)*hg/Lw/2
  Fcn3 : Fcn  Expr=m*g/4+u(1)*hg/(Lf+Lr)/2+u(2)*hg/Lw/2
  Fcn4 : Fcn  Expr=((-u(1)*hg+Lr*m*g)*(-u(2)*hg+m*g*Lw/2))/((Lf+Lr)*m*g*Lw)
  Fcn5 : Fcn  Expr=((-u(1)*hg+Lf*m*g)*(u(2)*hg+m*g*Lw/2))/((Lf+Lr)*m*g*Lw)
  Fcn6 : Fcn  Expr=((u(1)*hg+Lf*m*g)*(-u(2)*hg+m*g*Lw/2))/((Lf+Lr)*m*g*Lw)
  Fcn7 : Fcn  Expr=((u(1)*hg+Lr*m*g)*(u(2)*hg+m*g*Lw/2))/((Lf+Lr)*m*g*Lw)
  Mux : Mux  Inputs=2
  Scope : Scope  NumInputPorts=8
  FR vertical load [N] : Outport
  FL vertical load [N] : Outport  Port=2
  RR vertical load [N] : Outport  Port=3
  RL vertical load [N] : Outport  Port=4
  wires:
  Fy/1 -> Mux/2
  Fx/1 -> Mux/1
  Fcn4/1 -> FR vertical load [N]/1, Scope/1
  Fcn5/1 -> FL vertical load [N]/1, Scope/3
  Fcn6/1 -> RR vertical load [N]/1, Scope/5
  Fcn7/1 -> RL vertical load [N]/1, Scope/7
  Fcn/1 -> Scope/2
  Fcn1/1 -> Scope/4
  Fcn2/1 -> Scope/6
  Fcn3/1 -> Scope/8
  Mux/1 -> Fcn4/1, Fcn5/1, Fcn6/1, Fcn7/1, Fcn3/1, Fcn2/1, Fcn1/1, Fcn/1

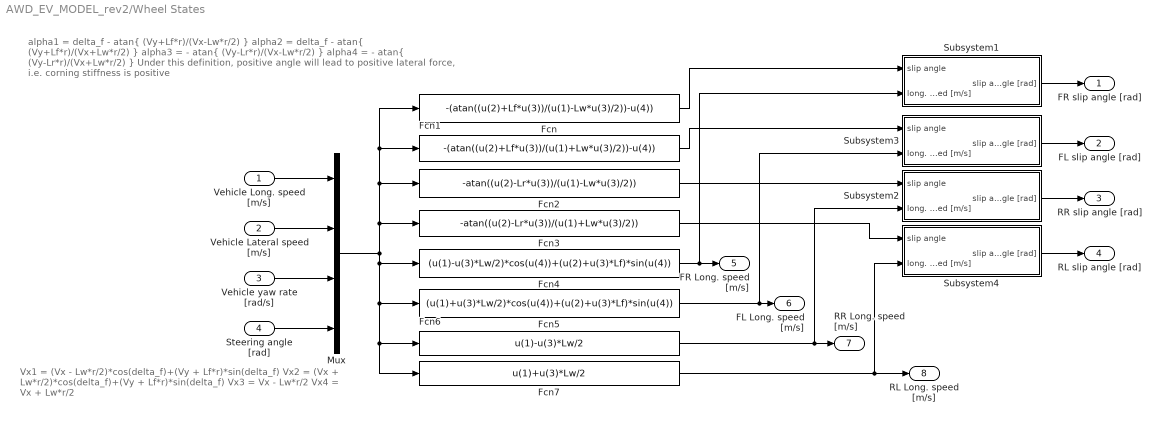
== system AWD_EV_MODEL_rev2/Wheel States ==
  note: alpha1 = delta_f - atan{ (Vy+Lf*r)/(Vx-Lw*r/2) }
      | alpha2 = delta_f - atan{ (Vy+Lf*r)/(Vx+Lw*r/2) }
      | alpha3 = - atan{ (Vy-Lr*r)/(Vx-Lw*r/2) }
      | alpha4 = - atan{ (Vy-Lr*r)/(Vx+Lw*r/2) }
      | Under this definition, positive angle will lead to  positive lateral force,
      | i.e. corning stiffness is positive
  note: Vx1 = (Vx - Lw*r/2)*cos(delta_f)+(Vy + Lf*r)*sin(delta_f)
      | Vx2 = (Vx + Lw*r/2)*cos(delta_f)+(Vy + Lf*r)*sin(delta_f)
      | Vx3 = Vx - Lw*r/2
      | Vx4 = Vx + Lw*r/2
  Vehicle Long. speed [m/s] : Inport
  Vehicle Lateral speed [m/s] : Inport  Port=2
  Vehicle yaw rate [rad/s] : Inport  Port=3
  Steering angle [rad] : Inport  Port=4
  Fcn : Fcn  Expr=-(atan((u(2)+Lf*u(3))/(u(1)-Lw*u(3)/2))-u(4))
  Fcn1 : Fcn  Expr=-(atan((u(2)+Lf*u(3))/(u(1)+Lw*u(3)/2))-u(4))
  Fcn2 : Fcn  Expr=-atan((u(2)-Lr*u(3))/(u(1)-Lw*u(3)/2))
  Fcn3 : Fcn  Expr=-atan((u(2)-Lr*u(3))/(u(1)+Lw*u(3)/2))
  Fcn4 : Fcn  Expr=(u(1)-u(3)*Lw/2)*cos(u(4))+(u(2)+u(3)*Lf)*sin(u(4))
  Fcn5 : Fcn  Expr=(u(1)+u(3)*Lw/2)*cos(u(4))+(u(2)+u(3)*Lf)*sin(u(4))
  Fcn6 : Fcn  Expr=u(1)-u(3)*Lw/2
  Fcn7 : Fcn  Expr=u(1)+u(3)*Lw/2
  Mux : Mux
  Subsystem1 : Subsystem
  Subsystem2 : Subsystem
  Subsystem3 : Subsystem
  Subsystem4 : Subsystem
  "FR slip angle [rad] " : Outport
  "FL slip angle [rad] " : Outport  Port=2
  "RR slip angle [rad] " : Outport  Port=3
  "RL slip angle [rad] " : Outport  Port=4
  FR Long. speed [m/s] : Outport  Port=5
  FL Long. speed [m/s] : Outport  Port=6
  RR Long. speed [m/s] : Outport  Port=7
  RL Long. speed [m/s] : Outport  Port=8
  wires:
  Vehicle yaw rate [rad/s]/1 -> Mux/3
  Vehicle Lateral speed [m/s]/1 -> Mux/2
  Vehicle Long. speed [m/s]/1 -> Mux/1
  Steering angle [rad]/1 -> Mux/4
  Fcn4/1 -> FR Long. speed [m/s]/1, Subsystem1/2(long. speed [m/s])
  Fcn5/1 -> FL Long. speed [m/s]/1, Subsystem3/2(long. speed [m/s])
  Fcn6/1 -> RR Long. speed [m/s]/1, Subsystem2/2(long. speed [m/s])
  Fcn7/1 -> RL Long. speed [m/s]/1, Subsystem4/2(long. speed [m/s])
  Mux/1 -> Fcn5/1, Fcn7/1, Fcn6/1, Fcn4/1, Fcn3/1, Fcn2/1, Fcn1/1, Fcn/1
  Subsystem1/1(slip angle [rad]) -> "FR slip angle [rad] "/1
  Fcn/1 -> Subsystem1/1(slip angle)
  Subsystem3/1(slip angle [rad]) -> "FL slip angle [rad] "/1
  Fcn1/1 -> Subsystem3/1(slip angle)
  Fcn2/1 -> Subsystem2/1(slip angle)
  Fcn3/1 -> Subsystem4/1(slip angle)
  Subsystem2/1(slip angle [rad]) -> "RR slip angle [rad] "/1
  Subsystem4/1(slip angle [rad]) -> "RL slip angle [rad] "/1

== system AWD_EV_MODEL_rev2/FL Tire Mode/Magic Formula ==
  Slip ratio : Inport
  Slip angle [rad] : Inport  Port=2
  Longitudinal Position : Inport  Port=3
  Magic Formula Condition 1 : Subsystem
  Magic Formula Condition 2 : Subsystem
  Long. friction coefficient : Outport
  Lat. friction coefficient : Outport  Port=2
  wires:
  Slip ratio/1 -> Magic Formula Condition 1/1(Slip ratio)
  Slip angle [rad]/1 -> Magic Formula Condition 1/2(Slip angle [rad])
  Magic Formula Condition 1/1(Long. friction coefficient) -> Long. friction coefficient/1
  Magic Formula Condition 1/2(Lat. friction coefficient) -> Lat. friction coefficient/1

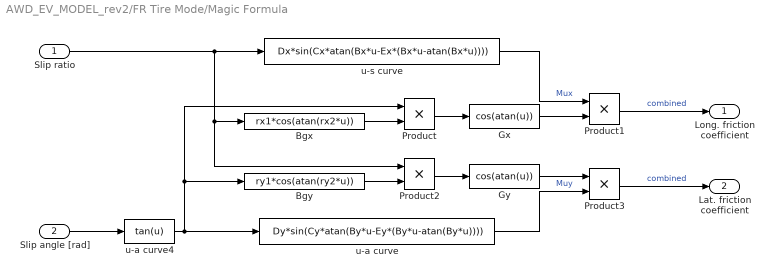
== system AWD_EV_MODEL_rev2/FR Tire Mode/Magic Formula ==
  Slip ratio : Inport
  Slip angle [rad] : Inport  Port=2
  Bgx : Fcn  Expr=rx1*cos(atan(rx2*u))
  Bgy : Fcn  Expr=ry1*cos(atan(ry2*u))
  Gx : Fcn  Expr=cos(atan(u))
  Gy : Fcn  Expr=cos(atan(u))
  Product{,1..3} (4 alike) : Product  RndMeth=Zero
  u-a curve : Fcn  Expr=Dy*sin(Cy*atan(By*u-Ey*(By*u-atan(By*u))))
  u-a curve4 : Fcn  Expr=tan(u)
  u-s curve : Fcn  Expr=Dx*sin(Cx*atan(Bx*u-Ex*(Bx*u-atan(Bx*u))))
  Long. friction coefficient : Outport
  Lat. friction coefficient : Outport  Port=2
  wires:
  Bgx/1 -> Product/2
  Bgy/1 -> Product2/2
  Slip angle [rad]/1 -> u-a curve4/1
  Product3/1 -> Lat. friction coefficient/1  "combined"
  Gy/1 -> Product3/1
  Product2/1 -> Gy/1
  Product1/1 -> Long. friction coefficient/1  "combined"
  Gx/1 -> Product1/2
  Product/1 -> Gx/1
  u-a curve4/1 -> Product/1, Bgy/1, u-a curve/1
  Slip ratio/1 -> Bgx/1, Product2/1, u-s curve/1
  u-a curve/1 -> Product3/2  "Muy"
  u-s curve/1 -> Product1/1  "Mux"

== system AWD_EV_MODEL_rev2/RL Tire Mode/Magic Formula ==
  Slip ratio : Inport
  Slip angle [rad] : Inport  Port=2
  Longitudinal Position : Inport  Port=3
  Magic Formula Condition 1 : Subsystem
  Long. friction coefficient : Outport
  Lat. friction coefficient : Outport  Port=2
  wires:
  Slip ratio/1 -> Magic Formula Condition 1/1(Slip ratio)
  Slip angle [rad]/1 -> Magic Formula Condition 1/2(Slip angle [rad])
  Magic Formula Condition 1/1(Long. friction coefficient) -> Long. friction coefficient/1
  Magic Formula Condition 1/2(Lat. friction coefficient) -> Lat. friction coefficient/1

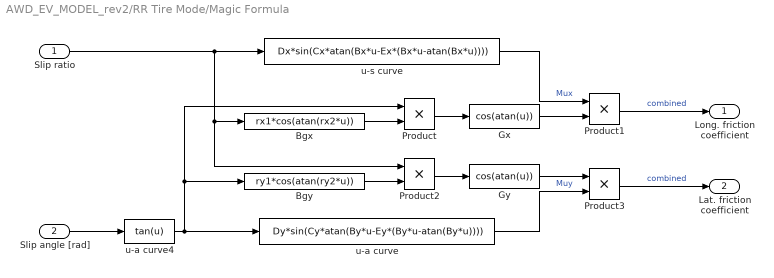
== system AWD_EV_MODEL_rev2/RR Tire Mode/Magic Formula ==
  Slip ratio : Inport
  Slip angle [rad] : Inport  Port=2
  Bgx : Fcn  Expr=rx1*cos(atan(rx2*u))
  Bgy : Fcn  Expr=ry1*cos(atan(ry2*u))
  Gx : Fcn  Expr=cos(atan(u))
  Gy : Fcn  Expr=cos(atan(u))
  Product{,1..3} (4 alike) : Product  RndMeth=Zero
  u-a curve : Fcn  Expr=Dy*sin(Cy*atan(By*u-Ey*(By*u-atan(By*u))))
  u-a curve4 : Fcn  Expr=tan(u)
  u-s curve : Fcn  Expr=Dx*sin(Cx*atan(Bx*u-Ex*(Bx*u-atan(Bx*u))))
  Long. friction coefficient : Outport
  Lat. friction coefficient : Outport  Port=2
  wires:
  Bgx/1 -> Product/2
  Bgy/1 -> Product2/2
  Slip angle [rad]/1 -> u-a curve4/1
  Product3/1 -> Lat. friction coefficient/1  "combined"
  Gy/1 -> Product3/1
  Product2/1 -> Gy/1
  Product1/1 -> Long. friction coefficient/1  "combined"
  Gx/1 -> Product1/2
  Product/1 -> Gx/1
  u-a curve4/1 -> Product/1, Bgy/1, u-a curve/1
  Slip ratio/1 -> Bgx/1, Product2/1, u-s curve/1
  u-a curve/1 -> Product3/2  "Muy"
  u-s curve/1 -> Product1/1  "Mux"

== system AWD_EV_MODEL_rev2/Wheel States/Subsystem1 ==
  slip angle : Inport
  long. speed [m/s] : Inport  Port=2
  If : If
  Merge1 : Merge
  negative slip angle : Subsystem  TreatAsAtomicUnit=on
  positive slip angle : Subsystem  TreatAsAtomicUnit=on
  slip angle [rad] : Outport
  wires:
  If/2 -> negative slip angle/Action
  negative slip angle/1(-in) -> Merge1/2
  positive slip angle/1(+in) -> Merge1/1
  If/1 -> positive slip angle/Action
  long. speed [m/s]/1 -> If/1
  slip angle/1 -> negative slip angle/1(in), positive slip angle/1(in)
  Merge1/1 -> slip angle [rad]/1

== system AWD_EV_MODEL_rev2/Wheel States/Subsystem2 ==
  slip angle : Inport
  long. speed [m/s] : Inport  Port=2
  If : If
  Merge1 : Merge
  negative slip angle : Subsystem  TreatAsAtomicUnit=on
  positive slip angle : Subsystem  TreatAsAtomicUnit=on
  slip angle [rad] : Outport
  wires:
  Merge1/1 -> slip angle [rad]/1
  slip angle/1 -> positive slip angle/1(in), negative slip angle/1(in)
  long. speed [m/s]/1 -> If/1
  If/1 -> positive slip angle/Action
  positive slip angle/1(+in) -> Merge1/1
  negative slip angle/1(-in) -> Merge1/2
  If/2 -> negative slip angle/Action

== system AWD_EV_MODEL_rev2/Wheel States/Subsystem3 ==
  slip angle : Inport
  long. speed [m/s] : Inport  Port=2
  If : If
  Merge1 : Merge
  negative slip angle : Subsystem  TreatAsAtomicUnit=on
  positive slip angle : Subsystem  TreatAsAtomicUnit=on
  slip angle [rad] : Outport
  wires:
  Merge1/1 -> slip angle [rad]/1
  slip angle/1 -> positive slip angle/1(in), negative slip angle/1(in)
  long. speed [m/s]/1 -> If/1
  If/1 -> positive slip angle/Action
  positive slip angle/1(+in) -> Merge1/1
  negative slip angle/1(-in) -> Merge1/2
  If/2 -> negative slip angle/Action

== system AWD_EV_MODEL_rev2/Wheel States/Subsystem4 ==
  slip angle : Inport
  long. speed [m/s] : Inport  Port=2
  If : If
  Merge1 : Merge
  negative slip angle : Subsystem  TreatAsAtomicUnit=on
  positive slip angle : Subsystem  TreatAsAtomicUnit=on
  slip angle [rad] : Outport
  wires:
  If/2 -> negative slip angle/Action
  negative slip angle/1(-in) -> Merge1/2
  positive slip angle/1(+in) -> Merge1/1
  If/1 -> positive slip angle/Action
  long. speed [m/s]/1 -> If/1
  slip angle/1 -> negative slip angle/1(in), positive slip angle/1(in)
  Merge1/1 -> slip angle [rad]/1

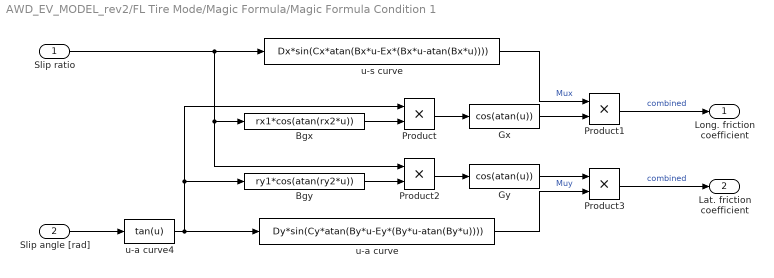
== system AWD_EV_MODEL_rev2/FL Tire Mode/Magic Formula/Magic Formula Condition 1 ==
  Slip ratio : Inport
  Slip angle [rad] : Inport  Port=2
  Bgx : Fcn  Expr=rx1*cos(atan(rx2*u))
  Bgy : Fcn  Expr=ry1*cos(atan(ry2*u))
  Gx : Fcn  Expr=cos(atan(u))
  Gy : Fcn  Expr=cos(atan(u))
  Product{,1..3} (4 alike) : Product  RndMeth=Zero
  u-a curve : Fcn  Expr=Dy*sin(Cy*atan(By*u-Ey*(By*u-atan(By*u))))
  u-a curve4 : Fcn  Expr=tan(u)
  u-s curve : Fcn  Expr=Dx*sin(Cx*atan(Bx*u-Ex*(Bx*u-atan(Bx*u))))
  Long. friction coefficient : Outport
  Lat. friction coefficient : Outport  Port=2
  wires:
  Bgx/1 -> Product/2
  Bgy/1 -> Product2/2
  Slip angle [rad]/1 -> u-a curve4/1
  Product3/1 -> Lat. friction coefficient/1  "combined"
  Gy/1 -> Product3/1
  Product2/1 -> Gy/1
  Product1/1 -> Long. friction coefficient/1  "combined"
  Gx/1 -> Product1/2
  Product/1 -> Gx/1
  u-a curve4/1 -> Product/1, Bgy/1, u-a curve/1
  Slip ratio/1 -> Bgx/1, Product2/1, u-s curve/1
  u-a curve/1 -> Product3/2  "Muy"
  u-s curve/1 -> Product1/1  "Mux"

== system AWD_EV_MODEL_rev2/FL Tire Mode/Magic Formula/Magic Formula Condition 2 ==
  Slip ratio : Inport
  Slip angle [rad] : Inport  Port=2
  Bgx : Fcn  Expr=rx1_2*cos(atan(rx2_2*u))
  Bgy : Fcn  Expr=ry1_2*cos(atan(ry2_2*u))
  Gx : Fcn  Expr=cos(atan(u))
  Gy : Fcn  Expr=cos(atan(u))
  Product{,1..3} (4 alike) : Product  RndMeth=Zero
  u-a curve : Fcn  Expr=Dy_2*sin(Cy_2*atan(By_2*u-Ey_2*(By_2*u-atan(By_2*u))))
  u-a curve4 : Fcn  Expr=tan(u)
  u-s curve : Fcn  Expr=Dx_2*sin(Cx_2*atan(Bx_2*u-Ex_2*(Bx_2*u-atan(Bx_2*u))))
  Long. friction coefficient : Outport
  Lat. friction coefficient : Outport  Port=2
  wires:
  Bgx/1 -> Product/2
  Bgy/1 -> Product2/2
  Slip angle [rad]/1 -> u-a curve4/1
  Product3/1 -> Lat. friction coefficient/1  "combined"
  Gy/1 -> Product3/1
  Product2/1 -> Gy/1
  Product1/1 -> Long. friction coefficient/1  "combined"
  Gx/1 -> Product1/2
  Product/1 -> Gx/1
  u-a curve4/1 -> Product/1, Bgy/1, u-a curve/1
  Slip ratio/1 -> Bgx/1, Product2/1, u-s curve/1
  u-a curve/1 -> Product3/2  "Muy"
  u-s curve/1 -> Product1/1  "Mux"

== system AWD_EV_MODEL_rev2/RL Tire Mode/Magic Formula/Magic Formula Condition 1 ==
  Slip ratio : Inport
  Slip angle [rad] : Inport  Port=2
  Bgx : Fcn  Expr=rx1*cos(atan(rx2*u))
  Bgy : Fcn  Expr=ry1*cos(atan(ry2*u))
  Gx : Fcn  Expr=cos(atan(u))
  Gy : Fcn  Expr=cos(atan(u))
  Product{,1..3} (4 alike) : Product  RndMeth=Zero
  u-a curve : Fcn  Expr=Dy*sin(Cy*atan(By*u-Ey*(By*u-atan(By*u))))
  u-a curve4 : Fcn  Expr=tan(u)
  u-s curve : Fcn  Expr=Dx*sin(Cx*atan(Bx*u-Ex*(Bx*u-atan(Bx*u))))
  Long. friction coefficient : Outport
  Lat. friction coefficient : Outport  Port=2
  wires:
  Bgx/1 -> Product/2
  Bgy/1 -> Product2/2
  Slip angle [rad]/1 -> u-a curve4/1
  Product3/1 -> Lat. friction coefficient/1  "combined"
  Gy/1 -> Product3/1
  Product2/1 -> Gy/1
  Product1/1 -> Long. friction coefficient/1  "combined"
  Gx/1 -> Product1/2
  Product/1 -> Gx/1
  u-a curve4/1 -> Product/1, Bgy/1, u-a curve/1
  Slip ratio/1 -> Bgx/1, Product2/1, u-s curve/1
  u-a curve/1 -> Product3/2  "Muy"
  u-s curve/1 -> Product1/1  "Mux"

== system AWD_EV_MODEL_rev2/Wheel States/Subsystem1/negative slip angle ==
  in : Inport
  Action Port : ActionPort  ActionType=else
  Gain : Gain  Gain=-1
  -in : Outport
  wires:
  in/1 -> Gain/1
  Gain/1 -> -in/1

== system AWD_EV_MODEL_rev2/Wheel States/Subsystem1/positive slip angle ==
  in : Inport
  Action Port : ActionPort  ActionType=then
  +in : Outport
  wires:
  in/1 -> +in/1

== system AWD_EV_MODEL_rev2/Wheel States/Subsystem2/negative slip angle ==
  in : Inport
  Action Port : ActionPort  ActionType=else
  Gain : Gain  Gain=-1
  -in : Outport
  wires:
  Gain/1 -> -in/1
  in/1 -> Gain/1

== system AWD_EV_MODEL_rev2/Wheel States/Subsystem2/positive slip angle ==
  in : Inport
  Action Port : ActionPort  ActionType=then
  +in : Outport
  wires:
  in/1 -> +in/1

== system AWD_EV_MODEL_rev2/Wheel States/Subsystem3/negative slip angle ==
  in : Inport
  Action Port : ActionPort  ActionType=else
  Gain : Gain  Gain=-1
  -in : Outport
  wires:
  Gain/1 -> -in/1
  in/1 -> Gain/1

== system AWD_EV_MODEL_rev2/Wheel States/Subsystem3/positive slip angle ==
  in : Inport
  Action Port : ActionPort  ActionType=then
  +in : Outport
  wires:
  in/1 -> +in/1

== system AWD_EV_MODEL_rev2/Wheel States/Subsystem4/negative slip angle ==
  in : Inport
  Action Port : ActionPort  ActionType=else
  Gain : Gain  Gain=-1
  -in : Outport
  wires:
  in/1 -> Gain/1
  Gain/1 -> -in/1

== system AWD_EV_MODEL_rev2/Wheel States/Subsystem4/positive slip angle ==
  in : Inport
  Action Port : ActionPort  ActionType=then
  +in : Outport
  wires:
  in/1 -> +in/1
